simulink model "Y_Model_20_Loads"  (R2018b)
settings: Solver=VariableStepAuto  StartTime=0.0  StopTime=sim_t  RelTol=1e-3
values from neighbouring files (symbols this model uses):
  dt = 5e-5    (= 5e-05)    [Y_multi_sim_loads.m]
  L = ones(num_sims, num_loads) * L_max    [Y_multi_sim_loads.m]
  P = rand(num_sims, num_loads) * (P_max - P_min) + P_min    [Y_multi_sim_loads.m]
  R = ones(num_sims, num_loads) * R_max    [Y_multi_sim_loads.m]
libraries: powerlib x270, powerlib_meascontrol x56
(part 1 of 4)
settings Model: Creator=mitchell  LastModifiedBy=mitchell

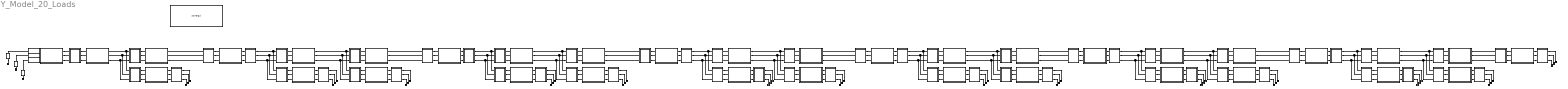
== system Y_Model_20_Loads ==
  AC Voltage Source : powerlib/Electrical Sources/AC Voltage Source  Amplitude=240  Phase=0  Frequency=50  SampleTime=0  Measurements=None  BusType=swing  Pref=10e3  Qref=0  Qmin=-inf  Qmax=+inf
  AC Voltage Source1 : powerlib/Electrical Sources/AC Voltage Source  Amplitude=240  Phase=-120  Frequency=50  SampleTime=0  Measurements=None  BusType=swing  Pref=10e3  Qref=0  Qmin=-inf  Qmax=+inf
  AC Voltage Source2 : powerlib/Electrical Sources/AC Voltage Source  Amplitude=240  Phase=-240  Frequency=50  SampleTime=0  Measurements=None  BusType=swing  Pref=10e3  Qref=0  Qmin=-inf  Qmax=+inf
  Load 1 : Subsystem
  Load 10 : Subsystem
  Load 11 : Subsystem
  Load 12 : Subsystem
  Load 13 : Subsystem
  Load 15 : Subsystem
  Load 16 : Subsystem
  Load 17 : Subsystem
  Load 18 : Subsystem
  Load 19 : Subsystem
  Load 2 : Subsystem
  Load 20 : Subsystem
  Load 21 : Subsystem
  Load 22 : Subsystem
  Load 24 : Subsystem
  Load 25 : Subsystem
  Load 26 : Subsystem
  Load 27 : Subsystem
  Load 28 : Subsystem
  Load 29 : Subsystem
  Load 3 : Subsystem
  Load 30 : Subsystem
  Load 31 : Subsystem
  Load 33 : Subsystem
  Load 34 : Subsystem
  Load 35 : Subsystem
  Load 36 : Subsystem
  Load 37 : Subsystem
  Load 38 : Subsystem
  Load 39 : Subsystem
  Load 4 : Subsystem
  Load 40 : Subsystem
  Load 42 : Subsystem
  Load 43 : Subsystem
  Load 44 : Subsystem
  Load 45 : Subsystem
  Load 46 : Subsystem
  Load 47 : Subsystem
  Load 48 : Subsystem
  Load 49 : Subsystem
  Load 5 : Subsystem
  Load 51 : Subsystem
  Load 52 : Subsystem
  Load 53 : Subsystem
  Load 54 : Subsystem
  Load 55 : Subsystem
  Load 56 : Subsystem
  Load 57 : Subsystem
  Load 58 : Subsystem
  Load 59 : Subsystem
  Load 60 : Subsystem
  Load 7 : Subsystem
  Load 8 : Subsystem
  Load 9 : Subsystem
  PMU 1 : Subsystem
  PMU 10 : Subsystem
  PMU 11 : Subsystem
  PMU 12 : Subsystem
  PMU 13 : Subsystem
  PMU 14 : Subsystem
  PMU 15 : Subsystem
  PMU 16 : Subsystem
  PMU 17 : Subsystem
  PMU 18 : Subsystem
  PMU 19 : Subsystem
  PMU 2 : Subsystem
  PMU 20 : Subsystem
  PMU 21 : Subsystem
  PMU 3 : Subsystem
  PMU 4 : Subsystem
  PMU 5 : Subsystem
  PMU 6 : Subsystem
  PMU 7 : Subsystem
  PMU 8 : Subsystem
  PMU 9 : Subsystem
  SCADA 1 : Subsystem
  SCADA 10 : Subsystem
  SCADA 11 : Subsystem
  SCADA 13 : Subsystem
  SCADA 14 : Subsystem
  SCADA 16 : Subsystem
  SCADA 17 : Subsystem
  SCADA 19 : Subsystem
  SCADA 2 : Subsystem
  SCADA 20 : Subsystem
  SCADA 4 : Subsystem
  SCADA 5 : Subsystem
  SCADA 7 : Subsystem
  SCADA 8 : Subsystem
  Series RLC Branch1 : powerlib/Elements/Series RLC Branch  LConnTagsString=__new0  RConnTagsString=__new0  BranchType=R  Resistance=1  Inductance=L(4)  SetiL0=off  InitialCurrent=0  Capacitance=0  Setx0=off  InitialVoltage=0  Measurements=None
  Series RLC Branch2 : powerlib/Elements/Series RLC Branch  LConnTagsString=__new0  RConnTagsString=__new0  BranchType=R  Resistance=1  Inductance=L(4)  SetiL0=off  InitialCurrent=0  Capacitance=0  Setx0=off  InitialVoltage=0  Measurements=None
  Series RLC Branch3 : powerlib/Elements/Series RLC Branch  LConnTagsString=__new0  RConnTagsString=__new0  BranchType=R  Resistance=1  Inductance=L(4)  SetiL0=off  InitialCurrent=0  Capacitance=0  Setx0=off  InitialVoltage=0  Measurements=None
  output Ground{1..7,11..13,17..22,26..33,37..42,46..51,55..63} (45 alike) : powerlib/Elements/Ground  LConnTagsString=a
      settings: SourceProductName=Simscape Electrical
  powergui1 : powerlib/powergui  Priority=1  SimulationMode=Discrete  SampleTime=dt  frequency=60  Iterations=500  frequencyindice=50  Pbase=100e6  ErrMax=0.0001  UnitsV=kV  UnitsW=MW  buscounter=1  FunctionMessages=off  echomessages=off  EnableUseOfTLC=off  CurrentSourceSwitches=off  DisableSnubberDevices=off  DisableRonSwitches=off  DisableVfSwitches=off  DisplayEquations=off  SolverType=Tustin/Backward Euler (TBE)  Interpol=off  ExternalGateDelay=off  methode=off  Ts=100  x0status=blocks  SPID=on  SwTol=0  HookPort=off  RestoreLinks=warning  ResistiveCurrentMeasurement=off  Frange=[0:2:500]  Ylog=off  Xlog=on  ShowGrid=off  save=off  variable=ZData  structure=0  ZoomFFT=off  StartTime=0.0  cycles=1  DisplayStyle=1  fundamental=60  FreqAxis=off  MaxFrequency=1000  frequencyindicesteady=1  RmsSteady=1  display=off
  connections:
  output Ground4/LConn1 -- AC Voltage Source2/LConn1
  output Ground27/LConn1 -- AC Voltage Source1/LConn1
  AC Voltage Source/LConn1 -- output Ground28/LConn1
  Series RLC Branch1/RConn1 -- PMU 1/LConn2
  Series RLC Branch2/RConn1 -- PMU 1/LConn3
  Load 3/LConn2 -- SCADA 1/RConn2 -- Load 1/LConn2
  Load 1/RConn1 -- SCADA 2/LConn1
  SCADA 2/LConn3 -- Load 1/RConn3
  AC Voltage Source2/RConn1 -- Series RLC Branch2/LConn1
  Series RLC Branch1/LConn1 -- AC Voltage Source1/RConn1
  Series RLC Branch3/LConn1 -- AC Voltage Source/RConn1
  PMU 1/LConn1 -- Series RLC Branch3/RConn1
  Load 1/LConn1 -- SCADA 1/RConn1 -- Load 3/LConn1
  PMU 1/RConn3 -- Load 2/LConn3
  PMU 1/RConn2 -- Load 2/LConn2
  PMU 1/RConn1 -- Load 2/LConn1
  Load 1/LConn3 -- SCADA 1/RConn3 -- Load 3/LConn3
  Load 2/RConn1 -- SCADA 1/LConn1
  Load 2/RConn2 -- SCADA 1/LConn2
  Load 2/RConn3 -- SCADA 1/LConn3
  Load 3/RConn1 -- PMU 2/LConn1
  Load 3/RConn2 -- PMU 2/LConn2
  Load 3/RConn3 -- PMU 2/LConn3
  PMU 2/RConn3 -- Load 5/LConn3
  PMU 2/RConn2 -- Load 5/LConn2
  PMU 2/RConn1 -- Load 5/LConn1
  Load 7/LConn2 -- SCADA 2/RConn2
  Load 7/LConn1 -- SCADA 2/RConn1
  SCADA 2/RConn3 -- Load 7/LConn3
  Load 7/RConn3 -- PMU 5/LConn3
  Load 7/RConn1 -- PMU 5/LConn1
  PMU 5/RConn2 -- Load 9/LConn2
  PMU 5/RConn1 -- Load 9/LConn1
  Load 7/RConn2 -- PMU 5/LConn2
  PMU 5/RConn3 -- Load 9/LConn3
  Load 1/RConn2 -- SCADA 2/LConn2
  Load 5/RConn2 -- output Ground6/LConn1
  Load 5/RConn1 -- output Ground5/LConn1
  Load 5/RConn3 -- output Ground7/LConn1
  Load 8/LConn2 -- Load 9/RConn2 -- Load 4/LConn2
  Load 4/LConn3 -- Load 9/RConn3 -- Load 8/LConn3
  Load 8/LConn1 -- Load 9/RConn1 -- Load 4/LConn1
  SCADA 4/LConn1 -- Load 4/RConn1
  Load 10/RConn3 -- output Ground1/LConn1
  Load 10/RConn2 -- output Ground3/LConn1
  SCADA 4/LConn3 -- Load 4/RConn3
  Load 10/RConn1 -- output Ground2/LConn1
  PMU 3/RConn2 -- Load 10/LConn2
  PMU 3/RConn3 -- Load 10/LConn3
  SCADA 4/LConn2 -- Load 4/RConn2
  Load 8/RConn1 -- PMU 3/LConn1
  PMU 3/RConn1 -- Load 10/LConn1
  Load 8/RConn2 -- PMU 3/LConn2
  Load 8/RConn3 -- PMU 3/LConn3
  Load 11/LConn1 -- SCADA 4/RConn1 -- Load 12/LConn1
  Load 12/LConn2 -- SCADA 4/RConn2 -- Load 11/LConn2
  Load 11/LConn3 -- SCADA 4/RConn3 -- Load 12/LConn3
  SCADA 5/LConn1 -- Load 11/RConn1
  Load 13/RConn3 -- output Ground11/LConn1
  Load 13/RConn2 -- output Ground13/LConn1
  SCADA 5/LConn3 -- Load 11/RConn3
  Load 13/RConn1 -- output Ground12/LConn1
  PMU 4/RConn2 -- Load 13/LConn2
  PMU 4/RConn3 -- Load 13/LConn3
  SCADA 5/LConn2 -- Load 11/RConn2
  Load 12/RConn1 -- PMU 4/LConn1
  PMU 4/RConn1 -- Load 13/LConn1
  Load 12/RConn2 -- PMU 4/LConn2
  Load 12/RConn3 -- PMU 4/LConn3
  Load 15/LConn1 -- SCADA 5/RConn1
  SCADA 5/RConn2 -- Load 15/LConn2
  SCADA 5/RConn3 -- Load 15/LConn3
  PMU 6/RConn2 -- Load 16/LConn2
  PMU 6/RConn3 -- Load 16/LConn3
  Load 15/RConn1 -- PMU 6/LConn1
  PMU 6/RConn1 -- Load 16/LConn1
  Load 15/RConn2 -- PMU 6/LConn2
  Load 15/RConn3 -- PMU 6/LConn3
  Load 16/RConn1 -- Load 17/LConn1 -- Load 18/LConn1
  Load 16/RConn2 -- Load 17/LConn2 -- Load 18/LConn2
  Load 16/RConn3 -- Load 18/LConn3 -- Load 17/LConn3
  SCADA 7/LConn1 -- Load 17/RConn1
  Load 19/RConn3 -- output Ground17/LConn1
  Load 19/RConn2 -- output Ground19/LConn1
  SCADA 7/LConn3 -- Load 17/RConn3
  Load 19/RConn1 -- output Ground18/LConn1
  PMU 7/RConn2 -- Load 19/LConn2
  PMU 7/RConn3 -- Load 19/LConn3
  SCADA 7/LConn2 -- Load 17/RConn2
  Load 18/RConn1 -- PMU 7/LConn1
  PMU 7/RConn1 -- Load 19/LConn1
  Load 18/RConn2 -- PMU 7/LConn2
  Load 18/RConn3 -- PMU 7/LConn3
  Load 20/LConn1 -- SCADA 7/RConn1 -- Load 21/LConn1
  Load 21/LConn2 -- SCADA 7/RConn2 -- Load 20/LConn2
  Load 20/LConn3 -- SCADA 7/RConn3 -- Load 21/LConn3
  SCADA 8/LConn1 -- Load 20/RConn1
  Load 22/RConn3 -- output Ground20/LConn1
  Load 22/RConn2 -- output Ground22/LConn1
  SCADA 8/LConn3 -- Load 20/RConn3
  Load 22/RConn1 -- output Ground21/LConn1
  PMU 8/RConn2 -- Load 22/LConn2
  PMU 8/RConn3 -- Load 22/LConn3
  SCADA 8/LConn2 -- Load 20/RConn2
  Load 21/RConn1 -- PMU 8/LConn1
  PMU 8/RConn1 -- Load 22/LConn1
  Load 21/RConn2 -- PMU 8/LConn2
  Load 21/RConn3 -- PMU 8/LConn3
  Load 24/LConn1 -- SCADA 8/RConn1
  SCADA 8/RConn2 -- Load 24/LConn2
  SCADA 8/RConn3 -- Load 24/LConn3
  PMU 9/RConn2 -- Load 25/LConn2
  PMU 9/RConn3 -- Load 25/LConn3
  Load 24/RConn1 -- PMU 9/LConn1
  PMU 9/RConn1 -- Load 25/LConn1
  Load 24/RConn2 -- PMU 9/LConn2
  Load 24/RConn3 -- PMU 9/LConn3
  Load 25/RConn1 -- Load 26/LConn1 -- Load 27/LConn1
  Load 25/RConn2 -- Load 26/LConn2 -- Load 27/LConn2
  Load 25/RConn3 -- Load 27/LConn3 -- Load 26/LConn3
  SCADA 10/LConn1 -- Load 26/RConn1
  Load 28/RConn3 -- output Ground26/LConn1
  Load 28/RConn2 -- output Ground30/LConn1
  SCADA 10/LConn3 -- Load 26/RConn3
  Load 28/RConn1 -- output Ground29/LConn1
  PMU 10/RConn2 -- Load 28/LConn2
  PMU 10/RConn3 -- Load 28/LConn3
  SCADA 10/LConn2 -- Load 26/RConn2
  Load 27/RConn1 -- PMU 10/LConn1
  PMU 10/RConn1 -- Load 28/LConn1
  Load 27/RConn2 -- PMU 10/LConn2
  Load 27/RConn3 -- PMU 10/LConn3
  Load 29/LConn1 -- SCADA 10/RConn1 -- Load 30/LConn1
  Load 30/LConn2 -- SCADA 10/RConn2 -- Load 29/LConn2
  Load 29/LConn3 -- SCADA 10/RConn3 -- Load 30/LConn3
  SCADA 11/LConn1 -- Load 29/RConn1
  Load 31/RConn3 -- output Ground31/LConn1
  Load 31/RConn2 -- output Ground33/LConn1
  SCADA 11/LConn3 -- Load 29/RConn3
  Load 31/RConn1 -- output Ground32/LConn1
  PMU 11/RConn2 -- Load 31/LConn2
  PMU 11/RConn3 -- Load 31/LConn3
  SCADA 11/LConn2 -- Load 29/RConn2
  Load 30/RConn1 -- PMU 11/LConn1
  PMU 11/RConn1 -- Load 31/LConn1
  Load 30/RConn2 -- PMU 11/LConn2
  Load 30/RConn3 -- PMU 11/LConn3
  Load 33/LConn1 -- SCADA 11/RConn1
  SCADA 11/RConn2 -- Load 33/LConn2
  SCADA 11/RConn3 -- Load 33/LConn3
  PMU 12/RConn2 -- Load 34/LConn2
  PMU 12/RConn3 -- Load 34/LConn3
  Load 33/RConn1 -- PMU 12/LConn1
  PMU 12/RConn1 -- Load 34/LConn1
  Load 33/RConn2 -- PMU 12/LConn2
  Load 33/RConn3 -- PMU 12/LConn3
  Load 34/RConn1 -- Load 35/LConn1 -- Load 36/LConn1
  Load 34/RConn2 -- Load 35/LConn2 -- Load 36/LConn2
  Load 34/RConn3 -- Load 35/LConn3 -- Load 36/LConn3
  SCADA 13/LConn1 -- Load 35/RConn1
  Load 37/RConn3 -- output Ground37/LConn1
  Load 37/RConn2 -- output Ground39/LConn1
  SCADA 13/LConn3 -- Load 35/RConn3
  Load 37/RConn1 -- output Ground38/LConn1
  PMU 13/RConn2 -- Load 37/LConn2
  PMU 13/RConn3 -- Load 37/LConn3
  SCADA 13/LConn2 -- Load 35/RConn2
  Load 36/RConn1 -- PMU 13/LConn1
  PMU 13/RConn1 -- Load 37/LConn1
  Load 36/RConn2 -- PMU 13/LConn2
  Load 36/RConn3 -- PMU 13/LConn3
  Load 38/LConn1 -- SCADA 13/RConn1 -- Load 39/LConn1
  Load 39/LConn2 -- SCADA 13/RConn2 -- Load 38/LConn2
  Load 38/LConn3 -- SCADA 13/RConn3 -- Load 39/LConn3
  SCADA 14/LConn1 -- Load 38/RConn1
  Load 40/RConn3 -- output Ground40/LConn1
  Load 40/RConn2 -- output Ground42/LConn1
  SCADA 14/LConn3 -- Load 38/RConn3
  Load 40/RConn1 -- output Ground41/LConn1
  PMU 14/RConn2 -- Load 40/LConn2
  PMU 14/RConn3 -- Load 40/LConn3
  SCADA 14/LConn2 -- Load 38/RConn2
  Load 39/RConn1 -- PMU 14/LConn1
  PMU 14/RConn1 -- Load 40/LConn1
  Load 39/RConn2 -- PMU 14/LConn2
  Load 39/RConn3 -- PMU 14/LConn3
  Load 42/LConn1 -- SCADA 14/RConn1
  SCADA 14/RConn2 -- Load 42/LConn2
  SCADA 14/RConn3 -- Load 42/LConn3
  PMU 15/RConn2 -- Load 43/LConn2
  PMU 15/RConn3 -- Load 43/LConn3
  Load 42/RConn1 -- PMU 15/LConn1
  PMU 15/RConn1 -- Load 43/LConn1
  Load 42/RConn2 -- PMU 15/LConn2
  Load 42/RConn3 -- PMU 15/LConn3
  Load 43/RConn1 -- Load 45/LConn1 -- Load 44/LConn1
  Load 43/RConn2 -- Load 45/LConn2 -- Load 44/LConn2
  Load 43/RConn3 -- Load 44/LConn3 -- Load 45/LConn3
  SCADA 16/LConn1 -- Load 44/RConn1
  Load 46/RConn3 -- output Ground46/LConn1
  Load 46/RConn2 -- output Ground48/LConn1
  SCADA 16/LConn3 -- Load 44/RConn3
  Load 46/RConn1 -- output Ground47/LConn1
  PMU 16/RConn2 -- Load 46/LConn2
  PMU 16/RConn3 -- Load 46/LConn3
  SCADA 16/LConn2 -- Load 44/RConn2
  Load 45/RConn1 -- PMU 16/LConn1
  PMU 16/RConn1 -- Load 46/LConn1
  Load 45/RConn2 -- PMU 16/LConn2
  Load 45/RConn3 -- PMU 16/LConn3
  Load 47/LConn1 -- SCADA 16/RConn1 -- Load 48/LConn1
  Load 48/LConn2 -- SCADA 16/RConn2 -- Load 47/LConn2
  Load 47/LConn3 -- SCADA 16/RConn3 -- Load 48/LConn3
  SCADA 17/LConn1 -- Load 47/RConn1
  Load 49/RConn3 -- output Ground49/LConn1
  Load 49/RConn2 -- output Ground51/LConn1
  SCADA 17/LConn3 -- Load 47/RConn3
  Load 49/RConn1 -- output Ground50/LConn1
  PMU 17/RConn2 -- Load 49/LConn2
  PMU 17/RConn3 -- Load 49/LConn3
  SCADA 17/LConn2 -- Load 47/RConn2
  Load 48/RConn1 -- PMU 17/LConn1
  PMU 17/RConn1 -- Load 49/LConn1
  Load 48/RConn2 -- PMU 17/LConn2
  Load 48/RConn3 -- PMU 17/LConn3
  Load 51/LConn1 -- SCADA 17/RConn1
  SCADA 17/RConn2 -- Load 51/LConn2
  SCADA 17/RConn3 -- Load 51/LConn3
  PMU 18/RConn2 -- Load 52/LConn2
  PMU 18/RConn3 -- Load 52/LConn3
  Load 51/RConn1 -- PMU 18/LConn1
  PMU 18/RConn1 -- Load 52/LConn1
  Load 51/RConn2 -- PMU 18/LConn2
  Load 51/RConn3 -- PMU 18/LConn3
  Load 52/RConn1 -- Load 53/LConn1 -- Load 54/LConn1
  Load 52/RConn2 -- Load 53/LConn2 -- Load 54/LConn2
  Load 52/RConn3 -- Load 54/LConn3 -- Load 53/LConn3
  SCADA 19/LConn1 -- Load 53/RConn1
  Load 55/RConn3 -- output Ground55/LConn1
  Load 55/RConn2 -- output Ground57/LConn1
  SCADA 19/LConn3 -- Load 53/RConn3
  Load 55/RConn1 -- output Ground56/LConn1
  PMU 19/RConn2 -- Load 55/LConn2
  PMU 19/RConn3 -- Load 55/LConn3
  SCADA 19/LConn2 -- Load 53/RConn2
  Load 54/RConn1 -- PMU 19/LConn1
  PMU 19/RConn1 -- Load 55/LConn1
  Load 54/RConn2 -- PMU 19/LConn2
  Load 54/RConn3 -- PMU 19/LConn3
  Load 56/LConn1 -- SCADA 19/RConn1 -- Load 57/LConn1
  Load 57/LConn2 -- SCADA 19/RConn2 -- Load 56/LConn2
  Load 56/LConn3 -- SCADA 19/RConn3 -- Load 57/LConn3
  SCADA 20/LConn1 -- Load 56/RConn1
  Load 58/RConn3 -- output Ground58/LConn1
  Load 58/RConn2 -- output Ground60/LConn1
  SCADA 20/LConn3 -- Load 56/RConn3
  Load 58/RConn1 -- output Ground59/LConn1
  PMU 20/RConn2 -- Load 58/LConn2
  PMU 20/RConn3 -- Load 58/LConn3
  SCADA 20/LConn2 -- Load 56/RConn2
  Load 57/RConn1 -- PMU 20/LConn1
  PMU 20/RConn1 -- Load 58/LConn1
  Load 57/RConn2 -- PMU 20/LConn2
  Load 57/RConn3 -- PMU 20/LConn3
  Load 60/RConn2 -- output Ground63/LConn1
  Load 59/RConn1 -- PMU 21/LConn1
  PMU 21/RConn2 -- Load 60/LConn2
  Load 60/RConn3 -- output Ground61/LConn1
  PMU 21/RConn1 -- Load 60/LConn1
  Load 60/RConn1 -- output Ground62/LConn1
  PMU 21/RConn3 -- Load 60/LConn3
  Load 59/RConn2 -- PMU 21/LConn2
  Load 59/RConn3 -- PMU 21/LConn3
  SCADA 20/RConn1 -- Load 59/LConn1
  SCADA 20/RConn2 -- Load 59/LConn2
  SCADA 20/RConn3 -- Load 59/LConn3

== system Y_Model_20_Loads/Load 1 ==
  Series RLC Branch3 : powerlib/Elements/Series RLC Branch  LConnTagsString=__new0  RConnTagsString=__new0  BranchType=RL  Resistance=R(1)  Inductance=L(1)  SetiL0=off  InitialCurrent=0  Capacitance=0  Setx0=off  InitialVoltage=0  Measurements=None
  Series RLC Branch4 : powerlib/Elements/Series RLC Branch  LConnTagsString=__new0  RConnTagsString=__new0  BranchType=RL  Resistance=R(1)  Inductance=L(1)  SetiL0=off  InitialCurrent=0  Capacitance=0  Setx0=off  InitialVoltage=0  Measurements=None
  Series RLC Branch5 : powerlib/Elements/Series RLC Branch  LConnTagsString=__new0  RConnTagsString=__new0  BranchType=RL  Resistance=R(1)  Inductance=L(1)  SetiL0=off  InitialCurrent=0  Capacitance=0  Setx0=off  InitialVoltage=0  Measurements=None
  Conn1 : PMIOPort  Side=Left
  Conn2 : PMIOPort  Port=2  Side=Right
  Conn3 : PMIOPort  Port=3  Side=Left
  Conn4 : PMIOPort  Port=4  Side=Right
  Conn5 : PMIOPort  Port=5  Side=Left
  Conn6 : PMIOPort  Port=6  Side=Right
  connections:
  Conn5/RConn1 -- Series RLC Branch5/LConn1
  Conn4/RConn1 -- Series RLC Branch4/RConn1
  Conn2/RConn1 -- Series RLC Branch3/RConn1
  Conn3/RConn1 -- Series RLC Branch4/LConn1
  Conn6/RConn1 -- Series RLC Branch5/RConn1
  Conn1/RConn1 -- Series RLC Branch3/LConn1

== system Y_Model_20_Loads/Load 10 ==
  Parallel RLC Load1 : powerlib/Elements/Parallel RLC Load  LConnTagsString=a  RConnTagsString=__new0  NominalVoltage=240  NominalFrequency=60  ActivePower=P(10)  InductivePower=P(10)/10  CapacitivePower=0  Setx0=off  InitialVoltage=0  SetiL0=off  InitialCurrent=0  Measurements=None  LoadType=constant Z
      settings: AttributesFormatString=\n  SourceProductName=Simscape Power Systems  SourceProductBaseCode=PS
  Parallel RLC Load2 : powerlib/Elements/Parallel RLC Load  LConnTagsString=a  RConnTagsString=__new0  NominalVoltage=240  NominalFrequency=60  ActivePower=P(10)  InductivePower=P(10)/10  CapacitivePower=0  Setx0=off  InitialVoltage=0  SetiL0=off  InitialCurrent=0  Measurements=None  LoadType=constant Z
      settings: AttributesFormatString=\n  SourceProductName=Simscape Power Systems  SourceProductBaseCode=PS
  Parallel RLC Load3 : powerlib/Elements/Parallel RLC Load  LConnTagsString=a  RConnTagsString=__new0  NominalVoltage=240  NominalFrequency=60  ActivePower=P(10)  InductivePower=P(10)/10  CapacitivePower=0  Setx0=off  InitialVoltage=0  SetiL0=off  InitialCurrent=0  Measurements=None  LoadType=constant Z
      settings: AttributesFormatString=\n  SourceProductName=Simscape Power Systems  SourceProductBaseCode=PS
  Conn1 : PMIOPort  Side=Left
  Conn2 : PMIOPort  Port=2  Side=Right
  Conn3 : PMIOPort  Port=3  Side=Left
  Conn4 : PMIOPort  Port=4  Side=Right
  Conn5 : PMIOPort  Port=5  Side=Left
  Conn6 : PMIOPort  Port=6  Side=Right
  connections:
  Parallel RLC Load3/LConn1 -- Conn5/RConn1
  Parallel RLC Load1/LConn1 -- Conn3/RConn1
  Parallel RLC Load2/LConn1 -- Conn1/RConn1
  Parallel RLC Load2/RConn1 -- Conn2/RConn1
  Parallel RLC Load1/RConn1 -- Conn4/RConn1
  Parallel RLC Load3/RConn1 -- Conn6/RConn1

== system Y_Model_20_Loads/Load 11 ==
  Series RLC Branch3 : powerlib/Elements/Series RLC Branch  LConnTagsString=__new0  RConnTagsString=__new0  BranchType=RL  Resistance=R(1)  Inductance=L(1)  SetiL0=off  InitialCurrent=0  Capacitance=0  Setx0=off  InitialVoltage=0  Measurements=None
  Series RLC Branch4 : powerlib/Elements/Series RLC Branch  LConnTagsString=__new0  RConnTagsString=__new0  BranchType=RL  Resistance=R(1)  Inductance=L(1)  SetiL0=off  InitialCurrent=0  Capacitance=0  Setx0=off  InitialVoltage=0  Measurements=None
  Series RLC Branch5 : powerlib/Elements/Series RLC Branch  LConnTagsString=__new0  RConnTagsString=__new0  BranchType=RL  Resistance=R(1)  Inductance=L(1)  SetiL0=off  InitialCurrent=0  Capacitance=0  Setx0=off  InitialVoltage=0  Measurements=None
  Conn1 : PMIOPort  Side=Left
  Conn2 : PMIOPort  Port=2  Side=Right
  Conn3 : PMIOPort  Port=3  Side=Left
  Conn4 : PMIOPort  Port=4  Side=Right
  Conn5 : PMIOPort  Port=5  Side=Left
  Conn6 : PMIOPort  Port=6  Side=Right
  connections:
  Conn5/RConn1 -- Series RLC Branch5/LConn1
  Conn4/RConn1 -- Series RLC Branch4/RConn1
  Conn2/RConn1 -- Series RLC Branch3/RConn1
  Conn3/RConn1 -- Series RLC Branch4/LConn1
  Conn6/RConn1 -- Series RLC Branch5/RConn1
  Conn1/RConn1 -- Series RLC Branch3/LConn1

== system Y_Model_20_Loads/Load 12 ==
  Series RLC Branch3 : powerlib/Elements/Series RLC Branch  LConnTagsString=__new0  RConnTagsString=__new0  BranchType=RL  Resistance=R(3)  Inductance=L(3)  SetiL0=off  InitialCurrent=0  Capacitance=0  Setx0=off  InitialVoltage=0  Measurements=None
  Series RLC Branch4 : powerlib/Elements/Series RLC Branch  LConnTagsString=__new0  RConnTagsString=__new0  BranchType=RL  Resistance=R(3)  Inductance=L(3)  SetiL0=off  InitialCurrent=0  Capacitance=0  Setx0=off  InitialVoltage=0  Measurements=None
  Series RLC Branch5 : powerlib/Elements/Series RLC Branch  LConnTagsString=__new0  RConnTagsString=__new0  BranchType=RL  Resistance=R(3)  Inductance=L(3)  SetiL0=off  InitialCurrent=0  Capacitance=0  Setx0=off  InitialVoltage=0  Measurements=None
  Conn1 : PMIOPort  Side=Left
  Conn2 : PMIOPort  Port=2  Side=Right
  Conn3 : PMIOPort  Port=3  Side=Left
  Conn4 : PMIOPort  Port=4  Side=Right
  Conn5 : PMIOPort  Port=5  Side=Left
  Conn6 : PMIOPort  Port=6  Side=Right
  connections:
  Conn5/RConn1 -- Series RLC Branch5/LConn1
  Conn4/RConn1 -- Series RLC Branch4/RConn1
  Conn2/RConn1 -- Series RLC Branch3/RConn1
  Conn3/RConn1 -- Series RLC Branch4/LConn1
  Conn6/RConn1 -- Series RLC Branch5/RConn1
  Conn1/RConn1 -- Series RLC Branch3/LConn1

== system Y_Model_20_Loads/Load 13 ==
  Parallel RLC Load1 : powerlib/Elements/Parallel RLC Load  LConnTagsString=a  RConnTagsString=__new0  NominalVoltage=240  NominalFrequency=60  ActivePower=P(13)  InductivePower=P(13)/10  CapacitivePower=0  Setx0=off  InitialVoltage=0  SetiL0=off  InitialCurrent=0  Measurements=None  LoadType=constant Z
      settings: AttributesFormatString=\n  SourceProductName=Simscape Power Systems  SourceProductBaseCode=PS
  Parallel RLC Load2 : powerlib/Elements/Parallel RLC Load  LConnTagsString=a  RConnTagsString=__new0  NominalVoltage=240  NominalFrequency=60  ActivePower=P(13)  InductivePower=P(13)/10  CapacitivePower=0  Setx0=off  InitialVoltage=0  SetiL0=off  InitialCurrent=0  Measurements=None  LoadType=constant Z
      settings: AttributesFormatString=\n  SourceProductName=Simscape Power Systems  SourceProductBaseCode=PS
  Parallel RLC Load3 : powerlib/Elements/Parallel RLC Load  LConnTagsString=a  RConnTagsString=__new0  NominalVoltage=240  NominalFrequency=60  ActivePower=P(13)  InductivePower=P(13)/10  CapacitivePower=0  Setx0=off  InitialVoltage=0  SetiL0=off  InitialCurrent=0  Measurements=None  LoadType=constant Z
      settings: AttributesFormatString=\n  SourceProductName=Simscape Power Systems  SourceProductBaseCode=PS
  Conn1 : PMIOPort  Side=Left
  Conn2 : PMIOPort  Port=2  Side=Right
  Conn3 : PMIOPort  Port=3  Side=Left
  Conn4 : PMIOPort  Port=4  Side=Right
  Conn5 : PMIOPort  Port=5  Side=Left
  Conn6 : PMIOPort  Port=6  Side=Right
  connections:
  Parallel RLC Load2/LConn1 -- Conn1/RConn1
  Parallel RLC Load2/RConn1 -- Conn2/RConn1
  Parallel RLC Load3/RConn1 -- Conn6/RConn1
  Parallel RLC Load3/LConn1 -- Conn5/RConn1
  Conn3/RConn1 -- Parallel RLC Load1/LConn1
  Parallel RLC Load1/RConn1 -- Conn4/RConn1

== system Y_Model_20_Loads/Load 15 ==
  Series RLC Branch3 : powerlib/Elements/Series RLC Branch  LConnTagsString=__new0  RConnTagsString=__new0  BranchType=RL  Resistance=R(3)  Inductance=L(3)  SetiL0=off  InitialCurrent=0  Capacitance=0  Setx0=off  InitialVoltage=0  Measurements=None
  Series RLC Branch4 : powerlib/Elements/Series RLC Branch  LConnTagsString=__new0  RConnTagsString=__new0  BranchType=RL  Resistance=R(3)  Inductance=L(3)  SetiL0=off  InitialCurrent=0  Capacitance=0  Setx0=off  InitialVoltage=0  Measurements=None
  Series RLC Branch5 : powerlib/Elements/Series RLC Branch  LConnTagsString=__new0  RConnTagsString=__new0  BranchType=RL  Resistance=R(3)  Inductance=L(3)  SetiL0=off  InitialCurrent=0  Capacitance=0  Setx0=off  InitialVoltage=0  Measurements=None
  Conn1 : PMIOPort  Side=Left
  Conn2 : PMIOPort  Port=2  Side=Right
  Conn3 : PMIOPort  Port=3  Side=Left
  Conn4 : PMIOPort  Port=4  Side=Right
  Conn5 : PMIOPort  Port=5  Side=Left
  Conn6 : PMIOPort  Port=6  Side=Right
  connections:
  Conn5/RConn1 -- Series RLC Branch5/LConn1
  Conn4/RConn1 -- Series RLC Branch4/RConn1
  Conn2/RConn1 -- Series RLC Branch3/RConn1
  Conn3/RConn1 -- Series RLC Branch4/LConn1
  Conn6/RConn1 -- Series RLC Branch5/RConn1
  Conn1/RConn1 -- Series RLC Branch3/LConn1

== system Y_Model_20_Loads/Load 16 ==
  Series RLC Branch3 : powerlib/Elements/Series RLC Branch  LConnTagsString=__new0  RConnTagsString=__new0  BranchType=RL  Resistance=R(4)  Inductance=L(4)  SetiL0=off  InitialCurrent=0  Capacitance=0  Setx0=off  InitialVoltage=0  Measurements=None
  Series RLC Branch4 : powerlib/Elements/Series RLC Branch  LConnTagsString=__new0  RConnTagsString=__new0  BranchType=RL  Resistance=R(4)  Inductance=L(4)  SetiL0=off  InitialCurrent=0  Capacitance=0  Setx0=off  InitialVoltage=0  Measurements=None
  Series RLC Branch5 : powerlib/Elements/Series RLC Branch  LConnTagsString=__new0  RConnTagsString=__new0  BranchType=RL  Resistance=R(4)  Inductance=L(4)  SetiL0=off  InitialCurrent=0  Capacitance=0  Setx0=off  InitialVoltage=0  Measurements=None
  Conn1 : PMIOPort  Side=Left
  Conn2 : PMIOPort  Port=2  Side=Right
  Conn3 : PMIOPort  Port=3  Side=Left
  Conn4 : PMIOPort  Port=4  Side=Right
  Conn5 : PMIOPort  Port=5  Side=Left
  Conn6 : PMIOPort  Port=6  Side=Right
  connections:
  Conn5/RConn1 -- Series RLC Branch5/LConn1
  Conn4/RConn1 -- Series RLC Branch4/RConn1
  Conn2/RConn1 -- Series RLC Branch3/RConn1
  Conn3/RConn1 -- Series RLC Branch4/LConn1
  Conn6/RConn1 -- Series RLC Branch5/RConn1
  Conn1/RConn1 -- Series RLC Branch3/LConn1

== system Y_Model_20_Loads/Load 17 ==
  Series RLC Branch3 : powerlib/Elements/Series RLC Branch  LConnTagsString=__new0  RConnTagsString=__new0  BranchType=RL  Resistance=R(1)  Inductance=L(1)  SetiL0=off  InitialCurrent=0  Capacitance=0  Setx0=off  InitialVoltage=0  Measurements=None
  Series RLC Branch4 : powerlib/Elements/Series RLC Branch  LConnTagsString=__new0  RConnTagsString=__new0  BranchType=RL  Resistance=R(1)  Inductance=L(1)  SetiL0=off  InitialCurrent=0  Capacitance=0  Setx0=off  InitialVoltage=0  Measurements=None
  Series RLC Branch5 : powerlib/Elements/Series RLC Branch  LConnTagsString=__new0  RConnTagsString=__new0  BranchType=RL  Resistance=R(1)  Inductance=L(1)  SetiL0=off  InitialCurrent=0  Capacitance=0  Setx0=off  InitialVoltage=0  Measurements=None
  Conn1 : PMIOPort  Side=Left
  Conn2 : PMIOPort  Port=2  Side=Right
  Conn3 : PMIOPort  Port=3  Side=Left
  Conn4 : PMIOPort  Port=4  Side=Right
  Conn5 : PMIOPort  Port=5  Side=Left
  Conn6 : PMIOPort  Port=6  Side=Right
  connections:
  Conn5/RConn1 -- Series RLC Branch5/LConn1
  Conn4/RConn1 -- Series RLC Branch4/RConn1
  Conn2/RConn1 -- Series RLC Branch3/RConn1
  Conn3/RConn1 -- Series RLC Branch4/LConn1
  Conn6/RConn1 -- Series RLC Branch5/RConn1
  Conn1/RConn1 -- Series RLC Branch3/LConn1

== system Y_Model_20_Loads/Load 18 ==
  Series RLC Branch3 : powerlib/Elements/Series RLC Branch  LConnTagsString=__new0  RConnTagsString=__new0  BranchType=RL  Resistance=R(3)  Inductance=L(3)  SetiL0=off  InitialCurrent=0  Capacitance=0  Setx0=off  InitialVoltage=0  Measurements=None
  Series RLC Branch4 : powerlib/Elements/Series RLC Branch  LConnTagsString=__new0  RConnTagsString=__new0  BranchType=RL  Resistance=R(3)  Inductance=L(3)  SetiL0=off  InitialCurrent=0  Capacitance=0  Setx0=off  InitialVoltage=0  Measurements=None
  Series RLC Branch5 : powerlib/Elements/Series RLC Branch  LConnTagsString=__new0  RConnTagsString=__new0  BranchType=RL  Resistance=R(3)  Inductance=L(3)  SetiL0=off  InitialCurrent=0  Capacitance=0  Setx0=off  InitialVoltage=0  Measurements=None
  Conn1 : PMIOPort  Side=Left
  Conn2 : PMIOPort  Port=2  Side=Right
  Conn3 : PMIOPort  Port=3  Side=Left
  Conn4 : PMIOPort  Port=4  Side=Right
  Conn5 : PMIOPort  Port=5  Side=Left
  Conn6 : PMIOPort  Port=6  Side=Right
  connections:
  Conn5/RConn1 -- Series RLC Branch5/LConn1
  Conn4/RConn1 -- Series RLC Branch4/RConn1
  Conn2/RConn1 -- Series RLC Branch3/RConn1
  Conn3/RConn1 -- Series RLC Branch4/LConn1
  Conn6/RConn1 -- Series RLC Branch5/RConn1
  Conn1/RConn1 -- Series RLC Branch3/LConn1

== system Y_Model_20_Loads/Load 19 ==
  Parallel RLC Load1 : powerlib/Elements/Parallel RLC Load  LConnTagsString=a  RConnTagsString=__new0  NominalVoltage=240  NominalFrequency=60  ActivePower=P(19)  InductivePower=P(19)/10  CapacitivePower=0  Setx0=off  InitialVoltage=0  SetiL0=off  InitialCurrent=0  Measurements=None  LoadType=constant Z
      settings: AttributesFormatString=\n  SourceProductName=Simscape Power Systems  SourceProductBaseCode=PS
  Parallel RLC Load2 : powerlib/Elements/Parallel RLC Load  LConnTagsString=a  RConnTagsString=__new0  NominalVoltage=240  NominalFrequency=60  ActivePower=P(19)  InductivePower=P(19)/10  CapacitivePower=0  Setx0=off  InitialVoltage=0  SetiL0=off  InitialCurrent=0  Measurements=None  LoadType=constant Z
      settings: AttributesFormatString=\n  SourceProductName=Simscape Power Systems  SourceProductBaseCode=PS
  Parallel RLC Load3 : powerlib/Elements/Parallel RLC Load  LConnTagsString=a  RConnTagsString=__new0  NominalVoltage=240  NominalFrequency=60  ActivePower=P(19)  InductivePower=P(19)/10  CapacitivePower=0  Setx0=off  InitialVoltage=0  SetiL0=off  InitialCurrent=0  Measurements=None  LoadType=constant Z
      settings: AttributesFormatString=\n  SourceProductName=Simscape Power Systems  SourceProductBaseCode=PS
  Conn1 : PMIOPort  Side=Left
  Conn2 : PMIOPort  Port=2  Side=Right
  Conn3 : PMIOPort  Port=3  Side=Left
  Conn4 : PMIOPort  Port=4  Side=Right
  Conn5 : PMIOPort  Port=5  Side=Left
  Conn6 : PMIOPort  Port=6  Side=Right
  connections:
  Parallel RLC Load3/LConn1 -- Conn5/RConn1
  Parallel RLC Load1/RConn1 -- Conn4/RConn1
  Parallel RLC Load1/LConn1 -- Conn3/RConn1
  Parallel RLC Load2/LConn1 -- Conn1/RConn1
  Parallel RLC Load2/RConn1 -- Conn2/RConn1
  Parallel RLC Load3/RConn1 -- Conn6/RConn1

== system Y_Model_20_Loads/Load 2 ==
  Series RLC Branch3 : powerlib/Elements/Series RLC Branch  LConnTagsString=__new0  RConnTagsString=__new0  BranchType=RL  Resistance=R(2)  Inductance=L(2)  SetiL0=off  InitialCurrent=0  Capacitance=0  Setx0=off  InitialVoltage=0  Measurements=None
  Series RLC Branch4 : powerlib/Elements/Series RLC Branch  LConnTagsString=__new0  RConnTagsString=__new0  BranchType=RL  Resistance=R(2)  Inductance=L(2)  SetiL0=off  InitialCurrent=0  Capacitance=0  Setx0=off  InitialVoltage=0  Measurements=None
  Series RLC Branch5 : powerlib/Elements/Series RLC Branch  LConnTagsString=__new0  RConnTagsString=__new0  BranchType=RL  Resistance=R(2)  Inductance=L(2)  SetiL0=off  InitialCurrent=0  Capacitance=0  Setx0=off  InitialVoltage=0  Measurements=None
  Conn1 : PMIOPort  Side=Left
  Conn2 : PMIOPort  Port=2  Side=Right
  Conn3 : PMIOPort  Port=3  Side=Left
  Conn4 : PMIOPort  Port=4  Side=Right
  Conn5 : PMIOPort  Port=5  Side=Left
  Conn6 : PMIOPort  Port=6  Side=Right
  connections:
  Conn5/RConn1 -- Series RLC Branch5/LConn1
  Conn4/RConn1 -- Series RLC Branch4/RConn1
  Conn2/RConn1 -- Series RLC Branch3/RConn1
  Conn3/RConn1 -- Series RLC Branch4/LConn1
  Conn6/RConn1 -- Series RLC Branch5/RConn1
  Conn1/RConn1 -- Series RLC Branch3/LConn1

== system Y_Model_20_Loads/Load 20 ==
  Series RLC Branch3 : powerlib/Elements/Series RLC Branch  LConnTagsString=__new0  RConnTagsString=__new0  BranchType=RL  Resistance=R(1)  Inductance=L(1)  SetiL0=off  InitialCurrent=0  Capacitance=0  Setx0=off  InitialVoltage=0  Measurements=None
  Series RLC Branch4 : powerlib/Elements/Series RLC Branch  LConnTagsString=__new0  RConnTagsString=__new0  BranchType=RL  Resistance=R(1)  Inductance=L(1)  SetiL0=off  InitialCurrent=0  Capacitance=0  Setx0=off  InitialVoltage=0  Measurements=None
  Series RLC Branch5 : powerlib/Elements/Series RLC Branch  LConnTagsString=__new0  RConnTagsString=__new0  BranchType=RL  Resistance=R(1)  Inductance=L(1)  SetiL0=off  InitialCurrent=0  Capacitance=0  Setx0=off  InitialVoltage=0  Measurements=None
  Conn1 : PMIOPort  Side=Left
  Conn2 : PMIOPort  Port=2  Side=Right
  Conn3 : PMIOPort  Port=3  Side=Left
  Conn4 : PMIOPort  Port=4  Side=Right
  Conn5 : PMIOPort  Port=5  Side=Left
  Conn6 : PMIOPort  Port=6  Side=Right
  connections:
  Conn5/RConn1 -- Series RLC Branch5/LConn1
  Conn4/RConn1 -- Series RLC Branch4/RConn1
  Conn2/RConn1 -- Series RLC Branch3/RConn1
  Conn3/RConn1 -- Series RLC Branch4/LConn1
  Conn6/RConn1 -- Series RLC Branch5/RConn1
  Conn1/RConn1 -- Series RLC Branch3/LConn1

== system Y_Model_20_Loads/Load 21 ==
  Series RLC Branch3 : powerlib/Elements/Series RLC Branch  LConnTagsString=__new0  RConnTagsString=__new0  BranchType=RL  Resistance=R(3)  Inductance=L(3)  SetiL0=off  InitialCurrent=0  Capacitance=0  Setx0=off  InitialVoltage=0  Measurements=None
  Series RLC Branch4 : powerlib/Elements/Series RLC Branch  LConnTagsString=__new0  RConnTagsString=__new0  BranchType=RL  Resistance=R(3)  Inductance=L(3)  SetiL0=off  InitialCurrent=0  Capacitance=0  Setx0=off  InitialVoltage=0  Measurements=None
  Series RLC Branch5 : powerlib/Elements/Series RLC Branch  LConnTagsString=__new0  RConnTagsString=__new0  BranchType=RL  Resistance=R(3)  Inductance=L(3)  SetiL0=off  InitialCurrent=0  Capacitance=0  Setx0=off  InitialVoltage=0  Measurements=None
  Conn1 : PMIOPort  Side=Left
  Conn2 : PMIOPort  Port=2  Side=Right
  Conn3 : PMIOPort  Port=3  Side=Left
  Conn4 : PMIOPort  Port=4  Side=Right
  Conn5 : PMIOPort  Port=5  Side=Left
  Conn6 : PMIOPort  Port=6  Side=Right
  connections:
  Conn5/RConn1 -- Series RLC Branch5/LConn1
  Conn4/RConn1 -- Series RLC Branch4/RConn1
  Conn2/RConn1 -- Series RLC Branch3/RConn1
  Conn3/RConn1 -- Series RLC Branch4/LConn1
  Conn6/RConn1 -- Series RLC Branch5/RConn1
  Conn1/RConn1 -- Series RLC Branch3/LConn1

== system Y_Model_20_Loads/Load 22 ==
  Parallel RLC Load1 : powerlib/Elements/Parallel RLC Load  LConnTagsString=a  RConnTagsString=__new0  NominalVoltage=240  NominalFrequency=60  ActivePower=P(22)  InductivePower=P(22)/10  CapacitivePower=0  Setx0=off  InitialVoltage=0  SetiL0=off  InitialCurrent=0  Measurements=None  LoadType=constant Z
      settings: AttributesFormatString=\n  SourceProductName=Simscape Power Systems  SourceProductBaseCode=PS
  Parallel RLC Load2 : powerlib/Elements/Parallel RLC Load  LConnTagsString=a  RConnTagsString=__new0  NominalVoltage=240  NominalFrequency=60  ActivePower=P(22)  InductivePower=P(22)/10  CapacitivePower=0  Setx0=off  InitialVoltage=0  SetiL0=off  InitialCurrent=0  Measurements=None  LoadType=constant Z
      settings: AttributesFormatString=\n  SourceProductName=Simscape Power Systems  SourceProductBaseCode=PS
  Parallel RLC Load4 : powerlib/Elements/Parallel RLC Load  LConnTagsString=a  RConnTagsString=__new0  NominalVoltage=240  NominalFrequency=60  ActivePower=P(22)  InductivePower=P(22)/10  CapacitivePower=0  Setx0=off  InitialVoltage=0  SetiL0=off  InitialCurrent=0  Measurements=None  LoadType=constant Z
      settings: AttributesFormatString=\n  SourceProductName=Simscape Power Systems  SourceProductBaseCode=PS
  Conn1 : PMIOPort  Side=Left
  Conn2 : PMIOPort  Port=2  Side=Right
  Conn3 : PMIOPort  Port=3  Side=Left
  Conn4 : PMIOPort  Port=4  Side=Right
  Conn5 : PMIOPort  Port=5  Side=Left
  Conn6 : PMIOPort  Port=6  Side=Right
  connections:
  Parallel RLC Load4/LConn1 -- Conn1/RConn1
  Parallel RLC Load4/RConn1 -- Conn2/RConn1
  Parallel RLC Load1/LConn1 -- Conn3/RConn1
  Parallel RLC Load1/RConn1 -- Conn4/RConn1
  Parallel RLC Load2/LConn1 -- Conn5/RConn1
  Parallel RLC Load2/RConn1 -- Conn6/RConn1

== system Y_Model_20_Loads/Load 24 ==
  Series RLC Branch3 : powerlib/Elements/Series RLC Branch  LConnTagsString=__new0  RConnTagsString=__new0  BranchType=RL  Resistance=R(3)  Inductance=L(3)  SetiL0=off  InitialCurrent=0  Capacitance=0  Setx0=off  InitialVoltage=0  Measurements=None
  Series RLC Branch4 : powerlib/Elements/Series RLC Branch  LConnTagsString=__new0  RConnTagsString=__new0  BranchType=RL  Resistance=R(3)  Inductance=L(3)  SetiL0=off  InitialCurrent=0  Capacitance=0  Setx0=off  InitialVoltage=0  Measurements=None
  Series RLC Branch5 : powerlib/Elements/Series RLC Branch  LConnTagsString=__new0  RConnTagsString=__new0  BranchType=RL  Resistance=R(3)  Inductance=L(3)  SetiL0=off  InitialCurrent=0  Capacitance=0  Setx0=off  InitialVoltage=0  Measurements=None
  Conn1 : PMIOPort  Side=Left
  Conn2 : PMIOPort  Port=2  Side=Right
  Conn3 : PMIOPort  Port=3  Side=Left
  Conn4 : PMIOPort  Port=4  Side=Right
  Conn5 : PMIOPort  Port=5  Side=Left
  Conn6 : PMIOPort  Port=6  Side=Right
  connections:
  Conn5/RConn1 -- Series RLC Branch5/LConn1
  Conn4/RConn1 -- Series RLC Branch4/RConn1
  Conn2/RConn1 -- Series RLC Branch3/RConn1
  Conn3/RConn1 -- Series RLC Branch4/LConn1
  Conn6/RConn1 -- Series RLC Branch5/RConn1
  Conn1/RConn1 -- Series RLC Branch3/LConn1

== system Y_Model_20_Loads/Load 25 ==
  Series RLC Branch3 : powerlib/Elements/Series RLC Branch  LConnTagsString=__new0  RConnTagsString=__new0  BranchType=RL  Resistance=R(4)  Inductance=L(4)  SetiL0=off  InitialCurrent=0  Capacitance=0  Setx0=off  InitialVoltage=0  Measurements=None
  Series RLC Branch4 : powerlib/Elements/Series RLC Branch  LConnTagsString=__new0  RConnTagsString=__new0  BranchType=RL  Resistance=R(4)  Inductance=L(4)  SetiL0=off  InitialCurrent=0  Capacitance=0  Setx0=off  InitialVoltage=0  Measurements=None
  Series RLC Branch5 : powerlib/Elements/Series RLC Branch  LConnTagsString=__new0  RConnTagsString=__new0  BranchType=RL  Resistance=R(4)  Inductance=L(4)  SetiL0=off  InitialCurrent=0  Capacitance=0  Setx0=off  InitialVoltage=0  Measurements=None
  Conn1 : PMIOPort  Side=Left
  Conn2 : PMIOPort  Port=2  Side=Right
  Conn3 : PMIOPort  Port=3  Side=Left
  Conn4 : PMIOPort  Port=4  Side=Right
  Conn5 : PMIOPort  Port=5  Side=Left
  Conn6 : PMIOPort  Port=6  Side=Right
  connections:
  Conn5/RConn1 -- Series RLC Branch5/LConn1
  Conn4/RConn1 -- Series RLC Branch4/RConn1
  Conn2/RConn1 -- Series RLC Branch3/RConn1
  Conn3/RConn1 -- Series RLC Branch4/LConn1
  Conn6/RConn1 -- Series RLC Branch5/RConn1
  Conn1/RConn1 -- Series RLC Branch3/LConn1

== system Y_Model_20_Loads/Load 26 ==
  Series RLC Branch3 : powerlib/Elements/Series RLC Branch  LConnTagsString=__new0  RConnTagsString=__new0  BranchType=RL  Resistance=R(1)  Inductance=L(1)  SetiL0=off  InitialCurrent=0  Capacitance=0  Setx0=off  InitialVoltage=0  Measurements=None
  Series RLC Branch4 : powerlib/Elements/Series RLC Branch  LConnTagsString=__new0  RConnTagsString=__new0  BranchType=RL  Resistance=R(1)  Inductance=L(1)  SetiL0=off  InitialCurrent=0  Capacitance=0  Setx0=off  InitialVoltage=0  Measurements=None
  Series RLC Branch5 : powerlib/Elements/Series RLC Branch  LConnTagsString=__new0  RConnTagsString=__new0  BranchType=RL  Resistance=R(1)  Inductance=L(1)  SetiL0=off  InitialCurrent=0  Capacitance=0  Setx0=off  InitialVoltage=0  Measurements=None
  Conn1 : PMIOPort  Side=Left
  Conn2 : PMIOPort  Port=2  Side=Right
  Conn3 : PMIOPort  Port=3  Side=Left
  Conn4 : PMIOPort  Port=4  Side=Right
  Conn5 : PMIOPort  Port=5  Side=Left
  Conn6 : PMIOPort  Port=6  Side=Right
  connections:
  Conn5/RConn1 -- Series RLC Branch5/LConn1
  Conn4/RConn1 -- Series RLC Branch4/RConn1
  Conn2/RConn1 -- Series RLC Branch3/RConn1
  Conn3/RConn1 -- Series RLC Branch4/LConn1
  Conn6/RConn1 -- Series RLC Branch5/RConn1
  Conn1/RConn1 -- Series RLC Branch3/LConn1

== system Y_Model_20_Loads/Load 27 ==
  Series RLC Branch3 : powerlib/Elements/Series RLC Branch  LConnTagsString=__new0  RConnTagsString=__new0  BranchType=RL  Resistance=R(3)  Inductance=L(3)  SetiL0=off  InitialCurrent=0  Capacitance=0  Setx0=off  InitialVoltage=0  Measurements=None
  Series RLC Branch4 : powerlib/Elements/Series RLC Branch  LConnTagsString=__new0  RConnTagsString=__new0  BranchType=RL  Resistance=R(3)  Inductance=L(3)  SetiL0=off  InitialCurrent=0  Capacitance=0  Setx0=off  InitialVoltage=0  Measurements=None
  Series RLC Branch5 : powerlib/Elements/Series RLC Branch  LConnTagsString=__new0  RConnTagsString=__new0  BranchType=RL  Resistance=R(3)  Inductance=L(3)  SetiL0=off  InitialCurrent=0  Capacitance=0  Setx0=off  InitialVoltage=0  Measurements=None
  Conn1 : PMIOPort  Side=Left
  Conn2 : PMIOPort  Port=2  Side=Right
  Conn3 : PMIOPort  Port=3  Side=Left
  Conn4 : PMIOPort  Port=4  Side=Right
  Conn5 : PMIOPort  Port=5  Side=Left
  Conn6 : PMIOPort  Port=6  Side=Right
  connections:
  Conn5/RConn1 -- Series RLC Branch5/LConn1
  Conn4/RConn1 -- Series RLC Branch4/RConn1
  Conn2/RConn1 -- Series RLC Branch3/RConn1
  Conn3/RConn1 -- Series RLC Branch4/LConn1
  Conn6/RConn1 -- Series RLC Branch5/RConn1
  Conn1/RConn1 -- Series RLC Branch3/LConn1

== system Y_Model_20_Loads/Load 28 ==
  Parallel RLC Load1 : powerlib/Elements/Parallel RLC Load  LConnTagsString=a  RConnTagsString=__new0  NominalVoltage=240  NominalFrequency=60  ActivePower=P(28)  InductivePower=P(28)/10  CapacitivePower=0  Setx0=off  InitialVoltage=0  SetiL0=off  InitialCurrent=0  Measurements=None  LoadType=constant Z
      settings: AttributesFormatString=\n  SourceProductName=Simscape Power Systems  SourceProductBaseCode=PS
  Parallel RLC Load2 : powerlib/Elements/Parallel RLC Load  LConnTagsString=a  RConnTagsString=__new0  NominalVoltage=240  NominalFrequency=60  ActivePower=P(28)  InductivePower=P(28)/10  CapacitivePower=0  Setx0=off  InitialVoltage=0  SetiL0=off  InitialCurrent=0  Measurements=None  LoadType=constant Z
      settings: AttributesFormatString=\n  SourceProductName=Simscape Power Systems  SourceProductBaseCode=PS
  Parallel RLC Load3 : powerlib/Elements/Parallel RLC Load  LConnTagsString=a  RConnTagsString=__new0  NominalVoltage=240  NominalFrequency=60  ActivePower=P(28)  InductivePower=P(28)/10  CapacitivePower=0  Setx0=off  InitialVoltage=0  SetiL0=off  InitialCurrent=0  Measurements=None  LoadType=constant Z
      settings: AttributesFormatString=\n  SourceProductName=Simscape Power Systems  SourceProductBaseCode=PS
  Conn1 : PMIOPort  Side=Left
  Conn2 : PMIOPort  Port=2  Side=Right
  Conn3 : PMIOPort  Port=3  Side=Left
  Conn4 : PMIOPort  Port=4  Side=Right
  Conn5 : PMIOPort  Port=5  Side=Left
  Conn6 : PMIOPort  Port=6  Side=Right
  connections:
  Parallel RLC Load2/LConn1 -- Conn1/RConn1
  Parallel RLC Load2/RConn1 -- Conn2/RConn1
  Parallel RLC Load3/LConn1 -- Conn5/RConn1
  Parallel RLC Load3/RConn1 -- Conn6/RConn1
  Parallel RLC Load1/LConn1 -- Conn3/RConn1
  Parallel RLC Load1/RConn1 -- Conn4/RConn1

== system Y_Model_20_Loads/Load 29 ==
  Series RLC Branch3 : powerlib/Elements/Series RLC Branch  LConnTagsString=__new0  RConnTagsString=__new0  BranchType=RL  Resistance=R(1)  Inductance=L(1)  SetiL0=off  InitialCurrent=0  Capacitance=0  Setx0=off  InitialVoltage=0  Measurements=None
  Series RLC Branch4 : powerlib/Elements/Series RLC Branch  LConnTagsString=__new0  RConnTagsString=__new0  BranchType=RL  Resistance=R(1)  Inductance=L(1)  SetiL0=off  InitialCurrent=0  Capacitance=0  Setx0=off  InitialVoltage=0  Measurements=None
  Series RLC Branch5 : powerlib/Elements/Series RLC Branch  LConnTagsString=__new0  RConnTagsString=__new0  BranchType=RL  Resistance=R(1)  Inductance=L(1)  SetiL0=off  InitialCurrent=0  Capacitance=0  Setx0=off  InitialVoltage=0  Measurements=None
  Conn1 : PMIOPort  Side=Left
  Conn2 : PMIOPort  Port=2  Side=Right
  Conn3 : PMIOPort  Port=3  Side=Left
  Conn4 : PMIOPort  Port=4  Side=Right
  Conn5 : PMIOPort  Port=5  Side=Left
  Conn6 : PMIOPort  Port=6  Side=Right
  connections:
  Conn5/RConn1 -- Series RLC Branch5/LConn1
  Conn4/RConn1 -- Series RLC Branch4/RConn1
  Conn2/RConn1 -- Series RLC Branch3/RConn1
  Conn3/RConn1 -- Series RLC Branch4/LConn1
  Conn6/RConn1 -- Series RLC Branch5/RConn1
  Conn1/RConn1 -- Series RLC Branch3/LConn1

== system Y_Model_20_Loads/Load 3 ==
  Series RLC Branch3 : powerlib/Elements/Series RLC Branch  LConnTagsString=__new0  RConnTagsString=__new0  BranchType=RL  Resistance=R(3)  Inductance=L(3)  SetiL0=off  InitialCurrent=0  Capacitance=0  Setx0=off  InitialVoltage=0  Measurements=None
  Series RLC Branch4 : powerlib/Elements/Series RLC Branch  LConnTagsString=__new0  RConnTagsString=__new0  BranchType=RL  Resistance=R(3)  Inductance=L(3)  SetiL0=off  InitialCurrent=0  Capacitance=0  Setx0=off  InitialVoltage=0  Measurements=None
  Series RLC Branch5 : powerlib/Elements/Series RLC Branch  LConnTagsString=__new0  RConnTagsString=__new0  BranchType=RL  Resistance=R(3)  Inductance=L(3)  SetiL0=off  InitialCurrent=0  Capacitance=0  Setx0=off  InitialVoltage=0  Measurements=None
  Conn1 : PMIOPort  Side=Left
  Conn2 : PMIOPort  Port=2  Side=Right
  Conn3 : PMIOPort  Port=3  Side=Left
  Conn4 : PMIOPort  Port=4  Side=Right
  Conn5 : PMIOPort  Port=5  Side=Left
  Conn6 : PMIOPort  Port=6  Side=Right
  connections:
  Conn5/RConn1 -- Series RLC Branch5/LConn1
  Conn4/RConn1 -- Series RLC Branch4/RConn1
  Conn2/RConn1 -- Series RLC Branch3/RConn1
  Conn3/RConn1 -- Series RLC Branch4/LConn1
  Conn6/RConn1 -- Series RLC Branch5/RConn1
  Conn1/RConn1 -- Series RLC Branch3/LConn1

== system Y_Model_20_Loads/Load 30 ==
  Series RLC Branch3 : powerlib/Elements/Series RLC Branch  LConnTagsString=__new0  RConnTagsString=__new0  BranchType=RL  Resistance=R(3)  Inductance=L(3)  SetiL0=off  InitialCurrent=0  Capacitance=0  Setx0=off  InitialVoltage=0  Measurements=None
  Series RLC Branch4 : powerlib/Elements/Series RLC Branch  LConnTagsString=__new0  RConnTagsString=__new0  BranchType=RL  Resistance=R(3)  Inductance=L(3)  SetiL0=off  InitialCurrent=0  Capacitance=0  Setx0=off  InitialVoltage=0  Measurements=None
  Series RLC Branch5 : powerlib/Elements/Series RLC Branch  LConnTagsString=__new0  RConnTagsString=__new0  BranchType=RL  Resistance=R(3)  Inductance=L(3)  SetiL0=off  InitialCurrent=0  Capacitance=0  Setx0=off  InitialVoltage=0  Measurements=None
  Conn1 : PMIOPort  Side=Left
  Conn2 : PMIOPort  Port=2  Side=Right
  Conn3 : PMIOPort  Port=3  Side=Left
  Conn4 : PMIOPort  Port=4  Side=Right
  Conn5 : PMIOPort  Port=5  Side=Left
  Conn6 : PMIOPort  Port=6  Side=Right
  connections:
  Conn5/RConn1 -- Series RLC Branch5/LConn1
  Conn4/RConn1 -- Series RLC Branch4/RConn1
  Conn2/RConn1 -- Series RLC Branch3/RConn1
  Conn3/RConn1 -- Series RLC Branch4/LConn1
  Conn6/RConn1 -- Series RLC Branch5/RConn1
  Conn1/RConn1 -- Series RLC Branch3/LConn1

== system Y_Model_20_Loads/Load 31 ==
  Parallel RLC Load1 : powerlib/Elements/Parallel RLC Load  LConnTagsString=a  RConnTagsString=__new0  NominalVoltage=240  NominalFrequency=60  ActivePower=P(31)  InductivePower=P(31)/10  CapacitivePower=0  Setx0=off  InitialVoltage=0  SetiL0=off  InitialCurrent=0  Measurements=None  LoadType=constant Z
      settings: AttributesFormatString=\n  SourceProductName=Simscape Power Systems  SourceProductBaseCode=PS
  Parallel RLC Load2 : powerlib/Elements/Parallel RLC Load  LConnTagsString=a  RConnTagsString=__new0  NominalVoltage=240  NominalFrequency=60  ActivePower=P(31)  InductivePower=P(31)/10  CapacitivePower=0  Setx0=off  InitialVoltage=0  SetiL0=off  InitialCurrent=0  Measurements=None  LoadType=constant Z
      settings: AttributesFormatString=\n  SourceProductName=Simscape Power Systems  SourceProductBaseCode=PS
  Parallel RLC Load3 : powerlib/Elements/Parallel RLC Load  LConnTagsString=a  RConnTagsString=__new0  NominalVoltage=240  NominalFrequency=60  ActivePower=P(31)  InductivePower=P(31)/10  CapacitivePower=0  Setx0=off  InitialVoltage=0  SetiL0=off  InitialCurrent=0  Measurements=None  LoadType=constant Z
      settings: AttributesFormatString=\n  SourceProductName=Simscape Power Systems  SourceProductBaseCode=PS
  Conn1 : PMIOPort  Side=Left
  Conn2 : PMIOPort  Port=2  Side=Right
  Conn3 : PMIOPort  Port=3  Side=Left
  Conn4 : PMIOPort  Port=4  Side=Right
  Conn5 : PMIOPort  Port=5  Side=Left
  Conn6 : PMIOPort  Port=6  Side=Right
  connections:
  Parallel RLC Load1/LConn1 -- Conn3/RConn1
  Conn1/RConn1 -- Parallel RLC Load2/LConn1
  Parallel RLC Load2/RConn1 -- Conn2/RConn1
  Parallel RLC Load1/RConn1 -- Conn4/RConn1
  Parallel RLC Load3/RConn1 -- Conn6/RConn1
  Parallel RLC Load3/LConn1 -- Conn5/RConn1

== system Y_Model_20_Loads/Load 33 ==
  Series RLC Branch3 : powerlib/Elements/Series RLC Branch  LConnTagsString=__new0  RConnTagsString=__new0  BranchType=RL  Resistance=R(3)  Inductance=L(3)  SetiL0=off  InitialCurrent=0  Capacitance=0  Setx0=off  InitialVoltage=0  Measurements=None
  Series RLC Branch4 : powerlib/Elements/Series RLC Branch  LConnTagsString=__new0  RConnTagsString=__new0  BranchType=RL  Resistance=R(3)  Inductance=L(3)  SetiL0=off  InitialCurrent=0  Capacitance=0  Setx0=off  InitialVoltage=0  Measurements=None
  Series RLC Branch5 : powerlib/Elements/Series RLC Branch  LConnTagsString=__new0  RConnTagsString=__new0  BranchType=RL  Resistance=R(3)  Inductance=L(3)  SetiL0=off  InitialCurrent=0  Capacitance=0  Setx0=off  InitialVoltage=0  Measurements=None
  Conn1 : PMIOPort  Side=Left
  Conn2 : PMIOPort  Port=2  Side=Right
  Conn3 : PMIOPort  Port=3  Side=Left
  Conn4 : PMIOPort  Port=4  Side=Right
  Conn5 : PMIOPort  Port=5  Side=Left
  Conn6 : PMIOPort  Port=6  Side=Right
  connections:
  Conn5/RConn1 -- Series RLC Branch5/LConn1
  Conn4/RConn1 -- Series RLC Branch4/RConn1
  Conn2/RConn1 -- Series RLC Branch3/RConn1
  Conn3/RConn1 -- Series RLC Branch4/LConn1
  Conn6/RConn1 -- Series RLC Branch5/RConn1
  Conn1/RConn1 -- Series RLC Branch3/LConn1
